simulink model "B4SNSTest"  (R2023b)
settings: Solver=VariableStepAuto  StartTime=0.0  StopTime=40  RelTol=1E-4  AbsTol=1E-4
values from neighbouring files (symbols this model uses):
  Cm_B4 = 0.01    [B4.m]    (also in CtrlParaSNSTuning.m)
  EL_B4 = -60    [B4.m]    (also in CtrlParaSNSTuning.m)
  gL_B4 = 0.1    [B4.m]    (also in CtrlParaSNSTuning.m = 0.2008)
  V_B4_0 = -60    [B4.m]    (also in CtrlParaSNSTuning.m; InitPara.m)
  V_max_B4 = (43.3606 - 6.5761) / 2 + 6.5761    (= 24.96835)    [CtrlParaSNSTuning.m]
  V_min_B4 = 6.5761    [CtrlParaSNSTuning.m]
undefined symbols (not defined in the file or in its folder): Iapp
settings Model: SimulationMode=accelerator  Creator=liyan  LastModifiedBy=Yanjun
settings ModelReferenceCC: EnableRefExpFcnMdlSchedulingChecks=on

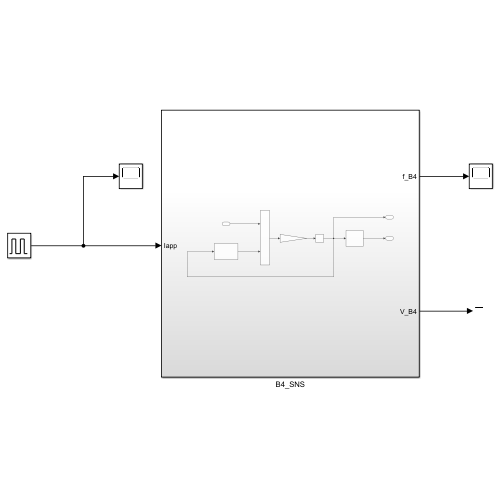
[thumbnail: Simulink's stored preview of the top-level diagram]
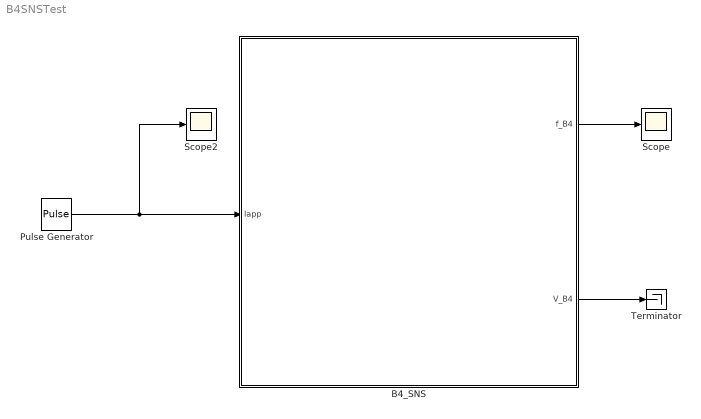
== system B4SNSTest ==
  B4_SNS : Subsystem
  Pulse Generator : DiscretePulseGenerator  PulseType=Time based  Amplitude=Iapp  Period=40  PulseWidth=0.3/40*100  PhaseDelay=30
  Scope : Scope
  Scope2 : Scope
  Terminator : Terminator
  wires:
  Pulse Generator/1 -> Scope2/1, B4_SNS/1(Iapp)
  B4_SNS/1(f_B4) -> Scope/1
  B4_SNS/2(V_B4) -> Terminator/1

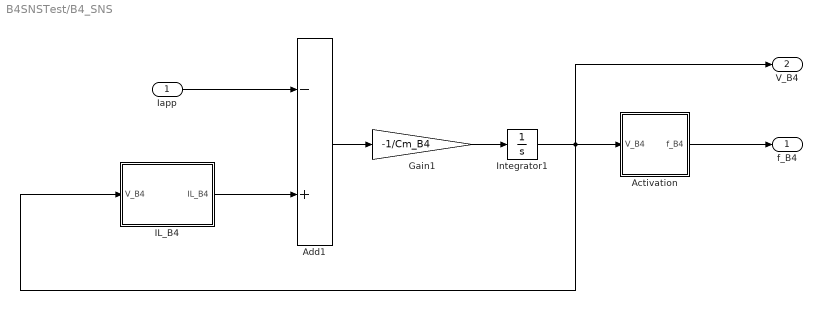
== system B4SNSTest/B4_SNS ==
  Iapp : Inport
  Activation : Subsystem
  Add1 : Sum  Inputs=-+
  Gain1 : Gain  Gain=-1/Cm_B4
  IL_B4 : Subsystem
  Integrator1 : Integrator  InitialCondition=V_B4_0
  f_B4 : Outport
  V_B4 : Outport  Port=2
  wires:
  Gain1/1 -> Integrator1/1
  Add1/1 -> Gain1/1
  Activation/1(f_B4) -> f_B4/1
  Integrator1/1 -> Activation/1(V_B4), IL_B4/1(V_B4), V_B4/1
  Iapp/1 -> Add1/1
  IL_B4/1(IL_B4) -> Add1/2

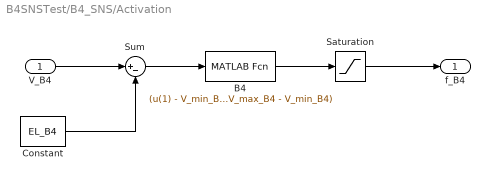
== system B4SNSTest/B4_SNS/Activation ==
  V_B4 : Inport
  B4 : MATLABFcn  MATLABFcn=(u(1) - V_min_B4)/(V_max_B4 - V_min_B4)
  Constant : Constant  Value=EL_B4
  Saturation : Saturate  UpperLimit=1  LowerLimit=0
  Sum : Sum  Inputs=|+-
  f_B4 : Outport
  wires:
  B4/1 -> Saturation/1
  Saturation/1 -> f_B4/1
  Sum/1 -> B4/1
  V_B4/1 -> Sum/1
  Constant/1 -> Sum/2

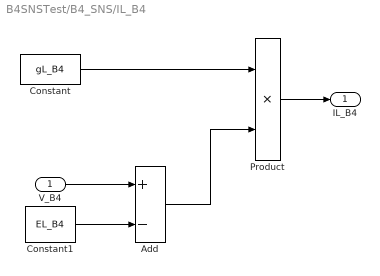
== system B4SNSTest/B4_SNS/IL_B4 ==
  V_B4 : Inport
  Add : Sum  Inputs=+-
  Constant : Constant  Value=gL_B4
  Constant1 : Constant  Value=EL_B4
  Product : Product
  IL_B4 : Outport
  wires:
  Constant1/1 -> Add/2
  V_B4/1 -> Add/1
  Constant/1 -> Product/1
  Add/1 -> Product/2
  Product/1 -> IL_B4/1
